simulink model "SingleTrack"  (Simulink 7.5)
settings: Solver=ode45  SolverMode=SingleTasking  StartTime=0.0  StopTime=inf  FixedStep=0.001  RelTol=1e-3
PreLoadFcn:
  | SingleTrack_params
undefined symbols (not defined in the file or in its folder): Car_Bdy1_mass, Car_Steering_i, Car_Whl_Radius, Car_WhlBaseF, Car_WhlBaseR, mEngineMax, PT_DL_iDiff, PT_GearBox_iForwardGears
libraries: CarMaker4SL x8, simulink x6
(part 4 of 4)

== system SingleTrack/CarMaker/Vehicle/User Vehicle (CM4SL)/CarAndTrailer/single-track mass point model/yaw/side forces ==
  vYaw : Inport  OutDataType=sfix(16)  OutScaling=2^0
  beta : Inport  Port=2  OutDataType=sfix(16)  OutScaling=2^0
  v : Inport  Port=3  OutDataType=sfix(16)  OutScaling=2^0
  StWhlAngle : Inport  Port=4  OutDataType=sfix(16)  OutScaling=2^0
  " " : Product  OutDataType=sfix(16)  OutScaling=2^0  SaturateOnIntegerOverflow=on  InputSameDT=on  OutDataTypeStr=Inherit: Same as first input
  "  " : Product  OutDataType=sfix(16)  OutScaling=2^0  SaturateOnIntegerOverflow=on  InputSameDT=on  OutDataTypeStr=Inherit: Same as first input
  "            " : Product  OutDataType=sfix(16)  OutScaling=2^0  SaturateOnIntegerOverflow=on  InputSameDT=on  OutDataTypeStr=Inherit: Same as first input
  "S_R * l_R " : Product  OutDataType=sfix(16)  OutScaling=2^0  SaturateOnIntegerOverflow=on  InputSameDT=on  OutDataTypeStr=Inherit: Same as first input
  "S_V * l_V " : Product  OutDataType=sfix(16)  OutScaling=2^0  SaturateOnIntegerOverflow=on  InputSameDT=on  OutDataTypeStr=Inherit: Same as first input
  Subsystem : Subsystem
  Sum : Sum  OutDataType=sfix(16)  OutScaling=2^0  SaturateOnIntegerOverflow=on  InputSameDT=on  OutDataTypeStr=Inherit: Same as first input
  Sum1 : Sum  Inputs=-+  OutDataType=sfix(16)  OutScaling=2^0  SaturateOnIntegerOverflow=on  InputSameDT=on  OutDataTypeStr=Inherit: Same as first input
  Sum4 : Sum  Inputs=+-  OutDataType=sfix(16)  OutScaling=2^0  SaturateOnIntegerOverflow=on  InputSameDT=on  OutDataTypeStr=Inherit: Same as first input
  c_alphaR : Gain  Gain=50000  ParameterDataType=sfix(16)  ParameterScaling=2^0  OutDataType=sfix(16)  OutScaling=2^0  SaturateOnIntegerOverflow=on  OutDataTypeStr=Inherit: Same as input  ParamDataTypeStr=Inherit: Same as input
  front wheel steering lock angle : Subsystem
  l__F : Constant  Value=Car_WhlBaseF  OutDataType=sfix(16)  OutScaling=2^0
  l__R : Constant  Value=-Car_WhlBaseR  OutDataType=sfix(16)  OutScaling=2^0
  S_F * l_F : Outport  OutDataType=sfix(16)  OutScaling=2^0
  S_R * l_R : Outport  Port=2  OutDataType=sfix(16)  OutScaling=2^0
  S_V : Outport  Port=3  OutDataType=sfix(16)  OutScaling=2^0
  S_R : Outport  Port=4  OutDataType=sfix(16)  OutScaling=2^0
  alpha_F : Outport  Port=5  OutDataType=sfix(16)  OutScaling=2^0
  alpha_R : Outport  Port=6  OutDataType=sfix(16)  OutScaling=2^0
  wires:
  beta/1 -> Sum1/1, Sum/1
  l__F/1 -> "  "/1, "S_V * l_V "/2
  Subsystem/1(vYaw/v) -> " "/1, "  "/2
  l__R/1 -> " "/2, "S_R * l_R "/2
  " "/1 -> Sum1/2
  "  "/1 -> Sum/2
  Sum1/1 -> c_alphaR/1, alpha_R/1
  c_alphaR/1 -> "S_R * l_R "/1, S_R/1
  "            "/1 -> "S_V * l_V "/1, S_V/1
  "S_V * l_V "/1 -> S_F * l_F/1
  vYaw/1 -> Subsystem/2(vYaw)
  v/1 -> Subsystem/1(v)
  Sum/1 -> Sum4/2, front wheel steering lock angle/2(beta + l_F * vYaw / v)
  front wheel steering lock angle/2(delta_F) -> Sum4/1
  Sum4/1 -> "            "/2, alpha_F/1
  "S_R * l_R "/1 -> S_R * l_R/1
  StWhlAngle/1 -> front wheel steering lock angle/1(StWhlAngle)
  front wheel steering lock angle/1(c_alphaF) -> "            "/1

== system SingleTrack/CarMaker/Vehicle/User Vehicle (CM4SL)/CarAndTrailer/single-track mass point model/yaw/sideslip angle ==
  vYaw : Inport  OutDataType=sfix(16)  OutScaling=2^0
  m : Inport  Port=2  OutDataType=sfix(16)  OutScaling=2^0
  v_dot : Inport  Port=3  OutDataType=sfix(16)  OutScaling=2^0
  v : Inport  Port=4  OutDataType=sfix(16)  OutScaling=2^0
  S : Inport  Port=5  OutDataType=sfix(16)  OutScaling=2^0
  " " : Product  Inputs=*/  OutDataType=sfix(16)  OutScaling=2^0  SaturateOnIntegerOverflow=on  InputSameDT=on  OutDataTypeStr=Inherit: Same as first input
  "  " : Product  OutDataType=sfix(16)  OutScaling=2^0  SaturateOnIntegerOverflow=on  InputSameDT=on  OutDataTypeStr=Inherit: Same as first input
  Subsystem : Subsystem
  Sum2 : Sum  Inputs=+-  OutDataType=sfix(16)  OutScaling=2^0  SaturateOnIntegerOverflow=on  InputSameDT=on  OutDataTypeStr=Inherit: Same as first input
  beta_dot * dt : Integrator  ExternalReset=level
  beta_dot : Outport  OutDataType=sfix(16)  OutScaling=2^0
  beta : Outport  Port=2  OutDataType=sfix(16)  OutScaling=2^0
  wires:
  [TRStart] -> beta_dot * dt/2
  beta_dot * dt/1 -> beta/1, "  "/2
  S/1 -> " "/1
  " "/1 -> Sum2/1
  v_dot/1 -> "  "/1
  m/1 -> " "/2
  "  "/1 -> Sum2/2
  Sum2/1 -> Subsystem/3(In3)
  vYaw/1 -> Subsystem/1(vYaw)
  Subsystem/1(Out1) -> beta_dot * dt/1, beta_dot/1
  v/1 -> Subsystem/2(v)

== system SingleTrack/CarMaker/Vehicle/User Vehicle (CM4SL)/CarAndTrailer/single-track mass point model/yaw/side forces/Subsystem ==
  v : Inport
  vYaw : Inport  Port=2
  If : If  IfExpression=u1 > 0.1 | u1 < -0.1
  If Action Subsystem : Subsystem  TreatAsAtomicUnit=on
  If Action Subsystem1 : Subsystem  TreatAsAtomicUnit=on
  Merge : Merge  InitialOutput=0
  vYaw/v : Outport
  wires:
  If Action Subsystem1/1(Out1) -> Merge/2
  If Action Subsystem/1(Out1) -> Merge/1
  Merge/1 -> vYaw/v/1
  If/2 -> If Action Subsystem1/Action
  If/1 -> If Action Subsystem/Action
  vYaw/1 -> If Action Subsystem/2(vYaw)
  v/1 -> If/1, If Action Subsystem/1(v)

== system SingleTrack/CarMaker/Vehicle/User Vehicle (CM4SL)/CarAndTrailer/single-track mass point model/yaw/side forces/front wheel steering lock angle ==
  StWhlAngle : Inport  OutDataType=sfix(16)  OutScaling=2^0
  beta + l_F * vYaw / v : Inport  Port=2  OutDataType=sfix(16)  OutScaling=2^0
  "   " : Product  OutDataType=sfix(16)  OutScaling=2^0  SaturateOnIntegerOverflow=on  InputSameDT=on  OutDataTypeStr=Inherit: Same as first input
  "     " : Constant  OutDataType=sfix(16)  OutScaling=2^0
  "      " : Product  Inputs=*/  OutDataType=sfix(16)  OutScaling=2^0  SaturateOnIntegerOverflow=on  InputSameDT=on  OutDataTypeStr=Inherit: Same as first input
  "       " : Product  Inputs=*/*  OutDataType=sfix(16)  OutScaling=2^0  SaturateOnIntegerOverflow=on  InputSameDT=on  OutDataTypeStr=Inherit: Same as first input
  1/ i_S : Gain  Gain=1/Car_Steering_i  ParameterDataType=sfix(16)  ParameterScaling=2^0  OutDataType=sfix(16)  OutScaling=2^0  SaturateOnIntegerOverflow=on  OutDataTypeStr=Inherit: Same as input  ParamDataTypeStr=Inherit: Same as input
  C_S : Constant  Value=10000  OutDataType=sfix(16)  OutScaling=2^0
  Sum2 : Sum  OutDataType=sfix(16)  OutScaling=2^0  SaturateOnIntegerOverflow=on  InputSameDT=on  OutDataTypeStr=Inherit: Same as first input
  Sum3 : Sum  OutDataType=sfix(16)  OutScaling=2^0  SaturateOnIntegerOverflow=on  InputSameDT=on  OutDataTypeStr=Inherit: Same as first input
  "c_alphaF " : Constant  Value=50000  OutDataType=sfix(16)  OutScaling=2^0
  n_F : Constant  Value=0.06  OutDataType=sfix(16)  OutScaling=2^0
  c_alphaF : Outport  OutDataType=sfix(16)  OutScaling=2^0
  delta_F : Outport  Port=2  OutDataType=sfix(16)  OutScaling=2^0
  wires:
  beta + l_F * vYaw / v/1 -> "   "/2
  "       "/1 -> Sum3/2, "   "/1
  StWhlAngle/1 -> 1/ i_S/1
  "   "/1 -> Sum2/2
  1/ i_S/1 -> Sum2/1
  "     "/1 -> Sum3/1
  Sum3/1 -> "      "/2
  Sum2/1 -> "      "/1
  C_S/1 -> "       "/2
  n_F/1 -> "       "/3
  "c_alphaF "/1 -> c_alphaF/1, "       "/1
  "      "/1 -> delta_F/1

== system SingleTrack/CarMaker/Vehicle/User Vehicle (CM4SL)/CarAndTrailer/single-track mass point model/yaw/sideslip angle/Subsystem ==
  vYaw : Inport
  v : Inport  Port=2
  In3 : Inport  Port=3
  If : If  IfExpression=u1 > 0.1 | u1 < -0.1
  If Action Subsystem : Subsystem  TreatAsAtomicUnit=on
  If Action Subsystem1 : Subsystem  TreatAsAtomicUnit=on
  Merge : Merge
  Sum1 : Sum  Inputs=-+  OutDataType=sfix(16)  OutScaling=2^0  SaturateOnIntegerOverflow=on  InputSameDT=on  OutDataTypeStr=Inherit: Same as first input
  Out1 : Outport
  wires:
  If/1 -> If Action Subsystem/Action
  In3/1 -> If Action Subsystem/2(In3)
  If/2 -> If Action Subsystem1/Action
  Merge/1 -> Sum1/2
  If Action Subsystem1/1(Out1) -> Merge/2
  If Action Subsystem/1(Out1) -> Merge/1
  Sum1/1 -> Out1/1
  v/1 -> If/1, If Action Subsystem/1(v)
  vYaw/1 -> Sum1/1

== system SingleTrack/CarMaker/Vehicle/User Vehicle (CM4SL)/CarAndTrailer/single-track mass point model/yaw/side forces/Subsystem/If Action Subsystem ==
  v : Inport
  vYaw : Inport  Port=2
  Action Port : ActionPort  ActionType=then
  vYaw / v : Product  Inputs=/*  OutDataType=sfix(16)  OutScaling=2^0  SaturateOnIntegerOverflow=on  InputSameDT=on  OutDataTypeStr=Inherit: Same as first input
  Out1 : Outport  OutDataType=sfix(16)  OutScaling=2^0  InitialOutput=0
  wires:
  vYaw / v/1 -> Out1/1
  vYaw/1 -> vYaw / v/2
  v/1 -> vYaw / v/1

== system SingleTrack/CarMaker/Vehicle/User Vehicle (CM4SL)/CarAndTrailer/single-track mass point model/yaw/side forces/Subsystem/If Action Subsystem1 ==
  Action Port : ActionPort  ActionType=else
  Constant : Constant  Value=0  OutDataType=sfix(16)  OutScaling=2^0
  Out1 : Outport  OutDataType=sfix(16)  OutScaling=2^0  InitialOutput=0
  wires:
  Constant/1 -> Out1/1

== system SingleTrack/CarMaker/Vehicle/User Vehicle (CM4SL)/CarAndTrailer/single-track mass point model/yaw/sideslip angle/Subsystem/If Action Subsystem ==
  v : Inport
  In3 : Inport  Port=2
  Action Port : ActionPort  ActionType=then
  "    " : Product  Inputs=/*  OutDataType=sfix(16)  OutScaling=2^0  SaturateOnIntegerOverflow=on  InputSameDT=on  OutDataTypeStr=Inherit: Same as first input
  Out1 : Outport  OutDataType=sfix(16)  OutScaling=2^0  InitialOutput=0
  wires:
  "    "/1 -> Out1/1
  In3/1 -> "    "/2
  v/1 -> "    "/1

== system SingleTrack/CarMaker/Vehicle/User Vehicle (CM4SL)/CarAndTrailer/single-track mass point model/yaw/sideslip angle/Subsystem/If Action Subsystem1 ==
  Action Port : ActionPort  ActionType=else
  Constant : Constant  Value=0  OutDataType=sfix(16)  OutScaling=2^0
  Out1 : Outport  OutDataType=sfix(16)  OutScaling=2^0  InitialOutput=0
  wires:
  Constant/1 -> Out1/1
